simulink model "angle"  (R2022a)
settings: Solver=FixedStepAuto  StartTime=0.0  StopTime=simulationtime  FixedStep=sampletime  RelTol=1e-3  EnableMultiTasking=on
InitFcn:
  | run("parametros.m")
StopFcn:
  | run("concatenacao.m")
  | sim('derivative',simulationtime)
values from neighbouring files (symbols this model uses):
  resol = 2*pi/400    (= 0.0157079632679)    [parametros.m]
libraries: arduinolib x2
settings Model: ExtModeTrigDuration=2  Creator=Franciele Sembay  LastModifiedBy=Franciele Sembay
settings OptimizationCC: EnhancedBackFolding=on  PassReuseOutputArgsAs=Individual arguments  ZeroExternalMemoryAtStartup=off  ZeroInternalMemoryAtStartup=off  MaxStackSize=64  OptimizeBlockOrder=speed  DifferentSizesBufferReuse=on  OptimizationCustomize=off  EfficientTunableParamExpr=on
settings DebuggingCC: ParameterTunabilityLossMsg=error
settings HardwareCC: ProdBitPerInt=16  ProdBitPerPointer=16  ProdBitPerSizeT=16  ProdBitPerPtrDiffT=16  ProdLargestAtomicFloat=None  ProdWordSize=8  ProdHWDeviceType=Atmel->AVR  UseEmbeddedCoderFeatures=off  UseSimulinkCoderFeatures=off
settings SFSimCC: MATLABDynamicMemAlloc=off
settings RTWCC: SystemTargetFile=ert.tlc  HardwareBoard=Arduino Uno  TemplateMakefile=ert_default_tmf  Toolchain=Arduino AVR  BuildConfiguration=Faster Runs
settings CodeAppCC: ForceParamTrailComments=on  IgnoreCustomStorageClasses=off  OperatorAnnotations=on  SimulinkDataObjDesc=on  SFDataObjDesc=on  InsertBlockDesc=on
settings ERTTargetCC: SupportContinuousTime=on  SupportNonInlinedSFcns=on  SupportVariableSizeSignals=on  ExtModeTransport=3  ExtModeStaticAlloc=on  ExtModeStaticAllocSize=250  ExtModeMexFile=ext_xcp  ExtModeIntrfLevel=Level2 - Open

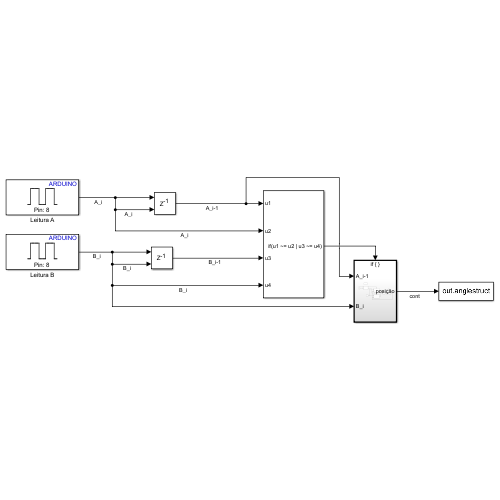
[thumbnail: Simulink's stored preview of the top-level diagram]
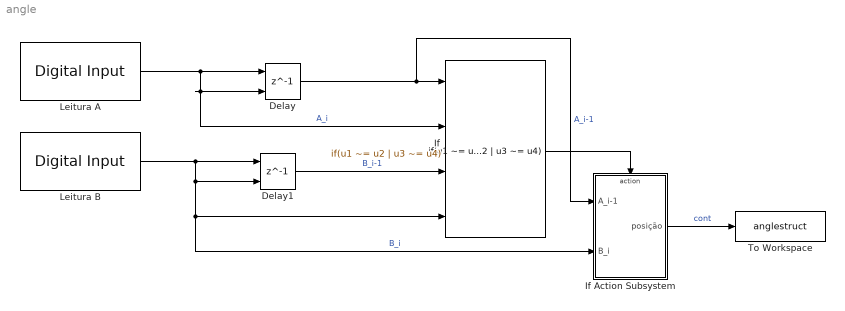
== system angle ==
  Delay : Delay  DelayLength=1  InitialConditionSource=Input port  InitialCondition=0
      settings: InputPortMap=u0,p4
  Delay1 : Delay  DelayLength=1  InitialConditionSource=Input port  InitialCondition=0
      settings: InputPortMap=u0,p4
  If : If  NumInputs=4  IfExpression=u1 ~= u2 | u3 ~= u4  ShowElse=off
  If Action Subsystem : Subsystem  TreatAsAtomicUnit=on
  Leitura A : arduinolib/Digital Input  pinNumber=pinoA  mode=Default  Direction=input  SampleTime=sampletime  blockPlatform=arduino
  Leitura B : arduinolib/Digital Input  pinNumber=pinoB  mode=Default  Direction=input  SampleTime=sampletime  blockPlatform=arduino
  To Workspace : ToWorkspace  VariableName=anglestruct  SaveFormat=Structure With Time  SampleTime=-1
  wires:
  Leitura A/1 -> Delay/1, Delay/2, If/2  "A_i"
  Delay/1 -> If Action Subsystem/1(A_i-1), If/1  "A_i-1"
  If Action Subsystem/1(posição) -> To Workspace/1  "cont"
  Delay1/1 -> If/3  "B_i-1"
  Leitura B/1 -> If Action Subsystem/2(B_i), If/4, Delay1/2, Delay1/1  "B_i"
  If/1 -> If Action Subsystem/Action

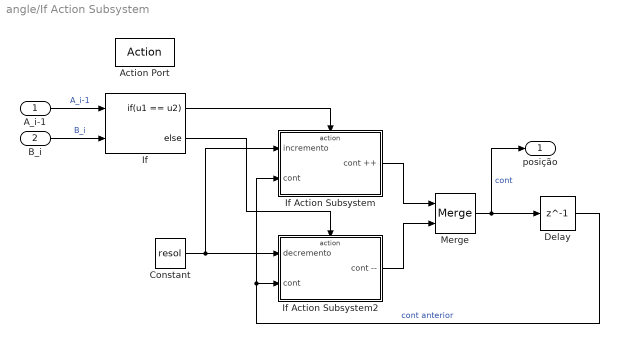
== system angle/If Action Subsystem ==
  A_i-1 : Inport
  B_i : Inport  Port=2
  Action Port : ActionPort  ActionPortLabel=if(u1 ~= u2 | u3 ~= u4)
  Constant : Constant  Value=resol
  Delay : Delay  DelayLength=1  InitialCondition=0
  If : If  NumInputs=2  IfExpression=u1 == u2
  If Action Subsystem : Subsystem  TreatAsAtomicUnit=on
  If Action Subsystem2 : Subsystem  TreatAsAtomicUnit=on
  Merge : Merge
  posição : Outport
  wires:
  A_i-1/1 -> If/1  "A_i-1"
  B_i/1 -> If/2  "B_i"
  If/1 -> If Action Subsystem/Action
  If/2 -> If Action Subsystem2/Action
  If Action Subsystem/1(cont ++) -> Merge/1
  If Action Subsystem2/1(cont --) -> Merge/2
  Merge/1 -> Delay/1, posição/1  "cont"
  Delay/1 -> If Action Subsystem/2(cont), If Action Subsystem2/2(cont)  "cont anterior"
  Constant/1 -> If Action Subsystem2/1(decremento), If Action Subsystem/1(incremento)

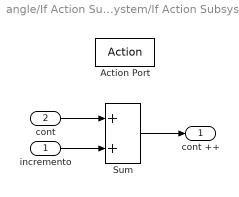
== system angle/If Action Subsystem/If Action Subsystem ==
  incremento : Inport
  cont : Inport  Port=2
  Action Port : ActionPort  ActionPortLabel=if(u1 ~= u2)
  Sum : Sum
  cont ++ : Outport
  wires:
  incremento/1 -> Sum/2
  Sum/1 -> cont ++/1
  cont/1 -> Sum/1

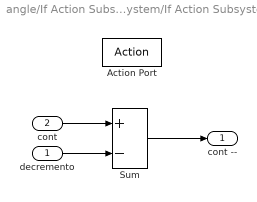
== system angle/If Action Subsystem/If Action Subsystem2 ==
  decremento : Inport
  cont : Inport  Port=2
  Action Port : ActionPort  ActionPortLabel=else
  Sum : Sum  Inputs=+-
  cont -- : Outport
  wires:
  decremento/1 -> Sum/2
  Sum/1 -> cont --/1
  cont/1 -> Sum/1
